simulink model "maintain_on_speed_harness_real"  (R2017b)
settings: Solver=VariableStepAuto  StartTime=0.0  StopTime=200  RelTol=1e-3
undefined symbols (not defined in the file): sigbuilder_block
settings Model: Creator=Kris  LastModifiedBy=Kris

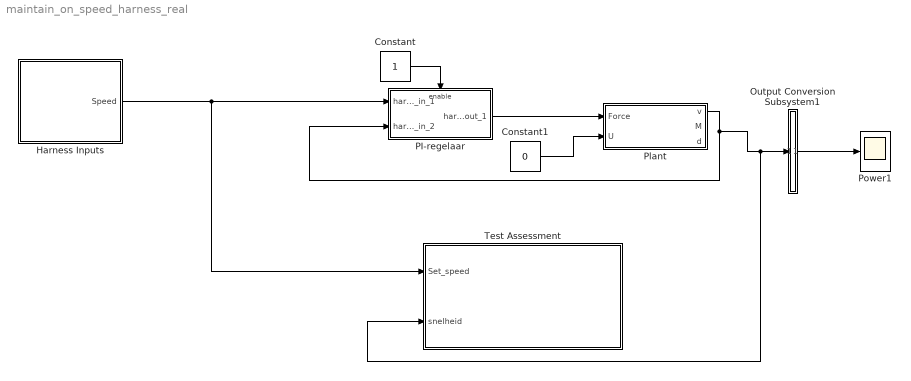
== system maintain_on_speed_harness_real ==
  Constant : Constant
  Constant1 : Constant  Value=0
  Harness Inputs : Subsystem  Tag=STV Subsys  LoadFcn=sigbuilder_block('load');  StartFcn=sigbuilder_block('start');  StopFcn=sigbuilder_block('stop');  ClipboardFcn=sigbuilder_block('clipboard');  mask(Sigbuilder block){tuvar=[0:10]}
      mask init:
      | if ~strcmp(get_param(bdroot(gcb),'SimulationStatus'),'stopped'),tuvar = sigbuilder_block('maskInit'); end
      settings: CopyFcn=sigbuilder_block('copy');  DeleteFcn=sigbuilder_block('delete');  ModelCloseFcn=sigbuilder_block('modelClose');  PreSaveFcn=sigbuilder_block('preSave');  PauseFcn=sigbuilder_block('pause');  ContinueFcn=sigbuilder_block('continue');  NameChangeFcn=sigbuilder_block('namechange');  OpenFcn=sigbuilder_block('open',[263.25 43.5 735.75 399.75 ]);  CloseFcn=sigbuilder_block('close');
      mask Display: plot(0, 0, 100, 100,[2, 2, 32, 32, 2], [68, 8, 8, 68, 68],[32, 2], [38, 38], [32, 19, 2],[53, 60, 44], [32, 17, 17, 2],[16, 16, 31, 31]);txt = getActiveGroup(gcbh);text(2, 100, txt,'verticalAlignment', 'top');
  Output Conversion Subsystem1 : Subsystem  Tag=__SLT_OCS__  Description=|
      | Signal spec.
      | and routing
      settings: AttributesFormatString=%<Description>
  "PI-regelaar " : Subsystem  Tag=__SL_testing_harness_stub_
  Plant : Subsystem
  Power1 : Scope
  Test Assessment : Test Sequence  TreatAsAtomicUnit=on
  wires:
  Plant/1(v) -> "PI-regelaar "/2(harness_in_2), Test Assessment/2(snelheid), Output Conversion Subsystem1/1(Inport_1)
  Output Conversion Subsystem1/1(Outport_1) -> Power1/1
  "PI-regelaar "/1(harness_out_1) -> Plant/1("Force ")
  Harness Inputs/1(Speed) -> Test Assessment/1(Set_speed), "PI-regelaar "/1(harness_in_1)
  Constant/1 -> "PI-regelaar "/Enable
  Constant1/1 -> Plant/2(U)

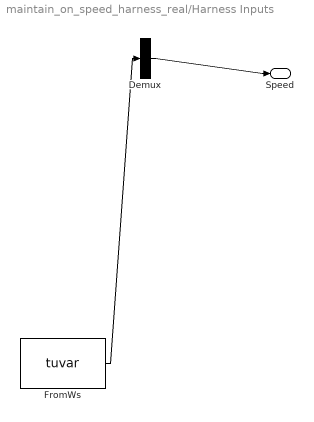
== system maintain_on_speed_harness_real/Harness Inputs ==
  Demux : Demux  Tag=STV Demux  Outputs=1
  FromWs : FromWorkspace  Tag=STV FromWs  VariableName=tuvar  SampleTime=0
      SigBuilderData=|
      | dataSet.timeRange = [0 180]
      | dataSet.name = 'Group 1'
      | sbobj.Name = 'Signal Builder'
      | sbobj.Groups.Name = 'Group 1'
      | sbobj.Groups.Signals.Name = 'Speed'
      | sbobj.Groups.Signals.XData = [0 41.4 41.4 76.6 76.6 114.8 114.8 147.8 147.8 180]
      | sbobj.Groups.Signals.YData = [50 50 12 12 50 50 30 30 40 40]
      | sbobj.Groups.TimeRange = [0 180]
  Speed : Outport  Tag=STV Outport
  wires:
  FromWs/1 -> Demux/1
  Demux/1 -> Speed/1

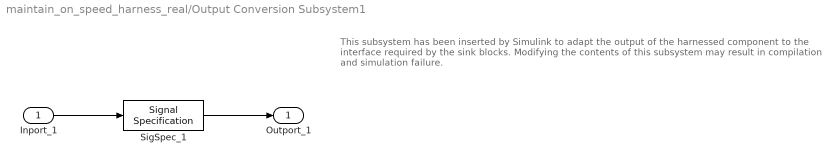
== system maintain_on_speed_harness_real/Output Conversion Subsystem1 ==
  note: This subsystem has been inserted by Simulink to adapt the output of the harnessed component to the interface required by the sink blocks.
      |  Modifying the contents of this subsystem may result in compilation and simulation failure.
  Inport_1 : Inport
  SigSpec_1 : SignalSpecification  OutDataTypeStr=double  Dimensions=[1]
  Outport_1 : Outport
  wires:
  Inport_1/1 -> SigSpec_1/1
  SigSpec_1/1 -> Outport_1/1

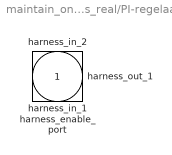
== system maintain_on_speed_harness_real/PI-regelaar  ==
  harness_in_1 : Inport
  harness_in_2 : Inport  Port=2
  harness_enable_port : EnablePort
  harness_out_1 : Outport

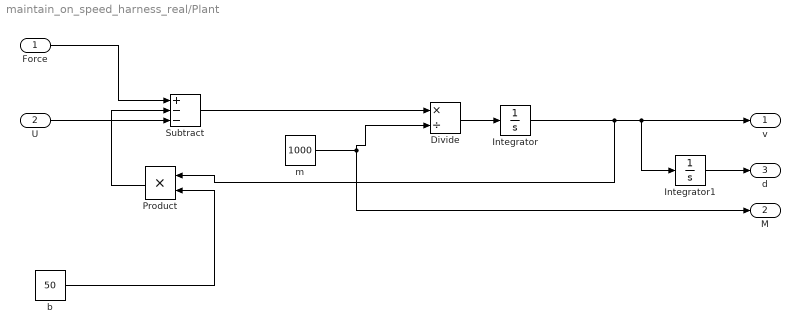
== system maintain_on_speed_harness_real/Plant ==
  "Force " : Inport
  U : Inport  Port=2
  Divide : Product  Inputs=*/
  Integrator : Integrator
  Integrator1 : Integrator
  Product : Product
  Subtract : Sum  Inputs=+--
  b : Constant  Value=50
  m : Constant  Value=1000
  v : Outport
  M : Outport  Port=2
  d : Outport  Port=3
  wires:
  Product/1 -> Subtract/2
  b/1 -> Product/2
  Subtract/1 -> Divide/1
  "Force "/1 -> Subtract/1
  Divide/1 -> Integrator/1
  m/1 -> Divide/2, M/1
  U/1 -> Subtract/3
  Integrator1/1 -> d/1
  Integrator/1 -> Product/1, v/1, Integrator1/1

== stateflow chart maintain_on_speed_harness_real/Test Assessment ==
  settings: stateMachineType=SIMPLIFIED_MACHINE
  state InitializeTest
    state step_1_1
      verify(Set_speed > (snelheid - (0.5/3.6)) && Set_speed < (snelheid +(0.5/3.6)));
    state step_1_2
    (default) -> (junction 22)
    InitializeTest -> (junction 22) [order 1]
    (junction 22) -> (junction 23) [order 1] : [t > 10
        | ]
    (junction 23) -> step_1_1 [order 1] : [~in(step_1_1)]
    (junction 22) -> (junction 56) [order 2]
    (junction 23) -> (junction 26) [order 2]
    (junction 56) -> (junction 57)
    (junction 57) -> step_1_2 [order 1] : [~in(step_1_2)]
    (junction 57) -> (junction 60) [order 2]
  state WaitStabilization
  (default) -> InitializeTest
  InitializeTest -> WaitStabilization [order 1] : [hasChanged(Set_speed)
      | ]
  WaitStabilization -> InitializeTest : [after(10,sec)
      | ]
  data: Set_speed input; snelheid input; speedtocheck local; speed local
